simulink model "rtl_sdr_fm"  (R2022b)
settings: Solver=VariableStepAuto  StartTime=0.0  StopTime=10  RelTol=1e-3
libraries: commanabbnd3 x1, dspfdesign x1, sdrrlib x1, dspvision x1
settings Model: Creator=tzajdel  LastModifiedBy=tzajdel
settings DebuggingCC: UnconnectedInputMsg=warning  UnconnectedOutputMsg=warning  UnconnectedLineMsg=warning
settings ModelReferenceCC: EnableRefExpFcnMdlSchedulingChecks=on
settings RTWCC: DLArmComputeVersion=19.05

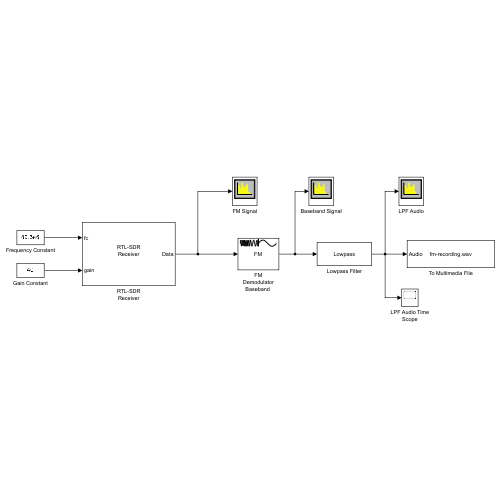
[thumbnail: Simulink's stored preview of the top-level diagram]
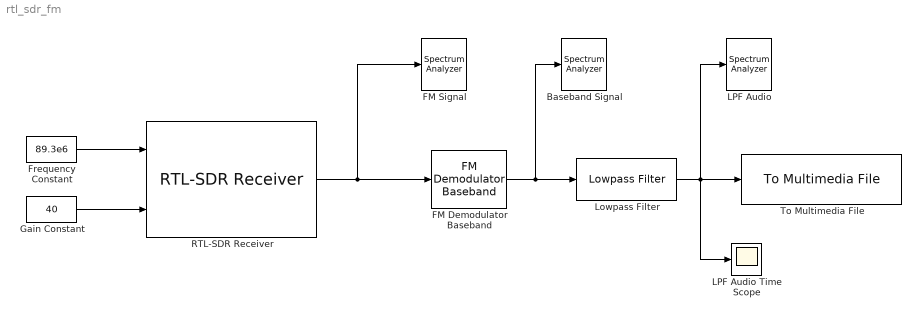
== system rtl_sdr_fm ==
  Baseband Signal : SpectrumAnalyzer
  "FM Demodulator Baseband " : commanabbnd3/FM Demodulator Baseband   FrequencyDeviation=75e3  SimulateUsing=Code generation
  FM Signal : SpectrumAnalyzer
  Frequency Constant : Constant  Value=89.3e6
  Gain Constant : Constant  Value=40
  LPF Audio : SpectrumAnalyzer
  LPF Audio Time Scope : Scope
  Lowpass Filter : dspfdesign/Lowpass Filter  FilterType=FIR  DesignForMinimumOrder=on  FilterOrder=50  PassbandFrequency=500  StopbandFrequency=1e3  PassbandRipple=0.1  StopbandAttenuation=80  InheritSampleRate=on  SampleRate=44100  SimulateUsing=Interpreted execution  roundingMode=Floor  coeffsDataTypeStr=fixdt(1,16)
  RTL-SDR Receiver : sdrrlib/RTL-SDR Receiver  IPAddress=0  CenterFrequencySource=Input port  CenterFrequency=89.3e6  GainSource=Input port  Gain=40  ADCRate=240e3  FrequencyCorrection=0  LostSamplesOutputPort=off  LatencyOutputPort=off  OutputDataType=single  FrameLength=10000  EnableBurstMode=off  NumFramesInBurst=20  sobjType=sdrr.internal.SDRRTLReceiverSL  dataUDPPort=-1  ctrlUDPPort=-1  subDeviceList=nosubdev  sdrBlockType=SDRBlockTypeSLT.SDRRxBlock  requester=UNUSED_BY_SFCN  sdrExecutionMode=SDRExecutionModeSLT.ExecModeHW  BypassUserLogic=off  DecimatorSelect=DDC decimator  SourceSelect=RF data  SineAmplitude=16000  EnableInternalClock=off  BypassIQBalance=off  IFBandwidth=40e6  ADCRateSource=Dialog  IntermediateFrequency=0  DecimationFactorSource=Dialog  DecimationFactor=512  RFFrequencyIsTunable=logical(1)  SampleTime=(10000)/(240e3)  IFBandwidthSource=Dialog  SineFrequency=30000  BypassDCBlockingFilter=off  IntermediateFrequencySource=Dialog  IQBalanceCoefficients=64  SkipAllHardwareResetAndInitialization=off  EnableIQCalibrationTable=on  CacheIQCalibrationTable=off  EnableOffsetTuning=off  EnableRTLAGC=off  EnableTestMode=off  EnableTunerAGC=off  FrequencyCorrectionSource=Dialog  NumMLBuffers=128  NumUSBBuffers=16  RTLCrystalFrequency=28800000  TunerCrystalFrequency=28800000
  To Multimedia File : dspvision/To Multimedia File  outputFilename=fm-recording.wav  streamSelection=Audio only  videoCompressor=None (uncompressed)  audioCompressor=None (uncompressed)  imagePorts=Separate color signals  fileType=WAV  audioDatatype=16-bit integer  fourcc=RGB  videoQuality=75  mj2000CompFactor=10
      settings: LibrarySourceBlock=dspsnks4/To Multimedia File
  wires:
  RTL-SDR Receiver/1 -> FM Signal/1, "FM Demodulator Baseband "/1
  Frequency Constant/1 -> RTL-SDR Receiver/1
  Gain Constant/1 -> RTL-SDR Receiver/2
  "FM Demodulator Baseband "/1 -> Lowpass Filter/1, Baseband Signal/1
  Lowpass Filter/1 -> To Multimedia File/1, LPF Audio Time Scope/1, LPF Audio/1
